simulink model "ex4"  (R2015b)
settings: Solver=VariableStepAuto  StartTime=0.0  StopTime=500.0  RelTol=1e-3
libraries: simulink x1
settings Model: Creator=ovi  LastModifiedBy=ovi

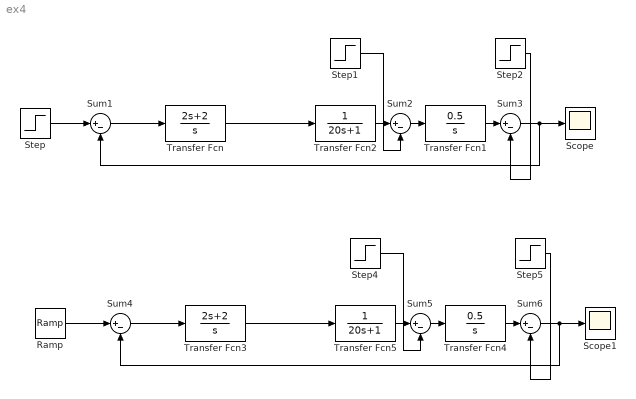
== system ex4 ==
  Ramp : simulink/Sources/Ramp  slope=1  start=0  X0=0
  Scope : Scope
  Scope1 : Scope
  Step : Step  SampleTime=0
  Step1 : Step  Time=3  After=0.2  SampleTime=0
  Step2 : Step  Time=6  After=0.1  SampleTime=0
  Step4 : Step  Time=3  After=0.2  SampleTime=0
  Step5 : Step  Time=6  After=0.1  SampleTime=0
  Sum{1..6} (6 alike) : Sum  Inputs=|+-
  Transfer Fcn : TransferFcn  Numerator=[2 2]  Denominator=[1 0]
  Transfer Fcn1 : TransferFcn  Numerator=[0.5]  Denominator=[1 0]
  Transfer Fcn2 : TransferFcn  Denominator=[20 1]
  Transfer Fcn3 : TransferFcn  Numerator=[2 2]  Denominator=[1 0]
  Transfer Fcn4 : TransferFcn  Numerator=[0.5]  Denominator=[1 0]
  Transfer Fcn5 : TransferFcn  Denominator=[20 1]
  wires:
  Transfer Fcn/1 -> Transfer Fcn2/1
  Transfer Fcn2/1 -> Sum2/1
  Sum2/1 -> Transfer Fcn1/1
  Step1/1 -> Sum2/2
  Step/1 -> Sum1/1
  Sum1/1 -> Transfer Fcn/1
  Transfer Fcn1/1 -> Sum3/1
  Sum3/1 -> Sum1/2, Scope/1
  Step2/1 -> Sum3/2
  Transfer Fcn3/1 -> Transfer Fcn5/1
  Transfer Fcn5/1 -> Sum5/1
  Sum5/1 -> Transfer Fcn4/1
  Step4/1 -> Sum5/2
  Ramp/1 -> Sum4/1
  Sum4/1 -> Transfer Fcn3/1
  Transfer Fcn4/1 -> Sum6/1
  Sum6/1 -> Sum4/2, Scope1/1
  Step5/1 -> Sum6/2
